simulink model "impedanceControl"  (R2014a)
settings: Solver=FixedStepDiscrete  StartTime=0.0  StopTime=Inf  FixedStep=Ts  RelTol=1e-3
InitFcn:
  | init_new_wbi_ID;
values from neighbouring files (symbols this model uses):
  Kd = 0.0001    [init_impedanceControl.m]    (also in init_new_wbi_ID.m)
  Kp = 1/10*diag( ones(1,ROBOT_DOF)  )    [init_impedanceControl.m]    (also in init_new_wbi_ID.m = 1/2*diag( ones(1,ROBOT_DOF)  ))
  ROBOT_DOF = 2    [init.m]    (also in init_get_q.m = 1; init_impedanceControl.m = 3; init_new_wbi_ID.m = 3)
libraries: WBCLibrary x11
settings Model: Creator=daniele  LastModifiedBy=daniele
settings DataIOCC: SignalLoggingSaveFormat=ModelDataLogs
settings DebuggingCC: MultiTaskDSMMsg=warning  MultiTaskCondExecSysMsg=none  StrictBusMsg=ErrorOnBusTreatedAsVector
settings RTWCC: IncludeERTFirstTime=on

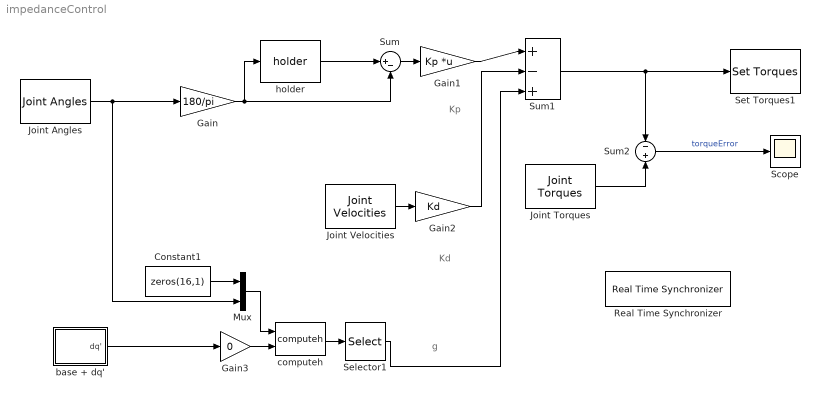
== system impedanceControl ==
  note: g
  note: Kd
  note: Kp
  Constant1 : Constant  Value=zeros(16,1)
  Gain : Gain  Gain=180/pi
  Gain1 : Gain  Gain=Kp  Multiplication=Matrix(K*u)
  Gain2 : Gain  Gain=Kd
  Gain3 : Gain  Gain=0
  Joint Angles : WBCLibrary/wholeBodyStates/Joint Angles  robotName=robotName  localName=localName
  Joint Torques : WBCLibrary/wholeBodyStates/Joint Torques  robotName=robotName  localName=localName
  Joint Velocities : WBCLibrary/wholeBodyStates/Joint Velocities  robotName=robotName  localName=localName
  Mux : Mux  Inputs=2
  Real Time Synchronizer : WBCLibrary/Utilities/Real Time Synchronizer  Priority=-10  threadPeriod=Ts
  Scope : Scope
      settings: ShowLegends=on
  Selector1 : Selector  InputPortWidth=ROBOT_DOF+6  Indices=[7:ROBOT_DOF+6]
  Set Torques1 : WBCLibrary/wholeBodyActuators/Set Torques  val=6  robotName=robotName  localName=localName
  Sum : Sum  Inputs=|+-
  Sum1 : Sum  Inputs=|+-+
  Sum2 : Sum  Inputs=-|+
  base + dq' : Subsystem
  computeh : WBCLibrary/wholeBodyModel/Dynamics/computeh  val=7  robotname=robotName  localname=localName
  "holder " : WBCLibrary/Utilities/holder 
  wires:
  Gain/1 -> Sum/2, "holder "/1
  "holder "/1 -> Sum/1
  Sum/1 -> Gain1/1
  Gain1/1 -> Sum1/1
  Joint Velocities/1 -> Gain2/1
  Gain2/1 -> Sum1/2
  Sum1/1 -> Sum2/1, Set Torques1/1
  Gain3/1 -> computeh/2
  base + dq'/1(dq') -> Gain3/1
  computeh/1 -> Selector1/1
  Mux/1 -> computeh/1
  Joint Angles/1 -> Mux/2, Gain/1
  Constant1/1 -> Mux/1
  Selector1/1 -> Sum1/3
  Sum2/1 -> Scope/1  "torqueError"
  Joint Torques/1 -> Sum2/2

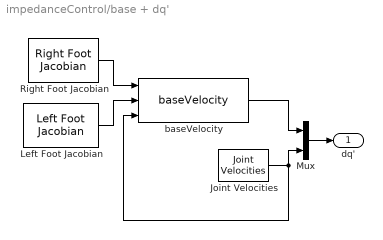
== system impedanceControl/base + dq' ==
  Joint Velocities : WBCLibrary/wholeBodyStates/Joint Velocities  robotName=robotName  localName=localName
  Left Foot Jacobian : WBCLibrary/wholeBodyModel/Jacobians/Left Foot Jacobian  robotName=robotName  localName=localName
  Mux : Mux  Inputs=2
  Right Foot Jacobian : WBCLibrary/wholeBodyModel/Jacobians/Right Foot Jacobian  robotName=robotName  localName=localName
  baseVelocity : WBCLibrary/Utilities/baseVelocity
  dq' : Outport
  wires:
  Left Foot Jacobian/1 -> baseVelocity/2
  Right Foot Jacobian/1 -> baseVelocity/1
  baseVelocity/1 -> Mux/1
  Joint Velocities/1 -> baseVelocity/3, Mux/2
  Mux/1 -> dq'/1
